simulink model "RainSnsrWiperMot_Method_1"  (R2021b)
settings: Solver=FixedStepDiscrete  StartTime=0.0  StopTime=10.0  FixedStep=0.01  RelTol=1e-3
undefined symbols (not defined in the file or in its folder): sigbuilder_block
libraries: simulink x1
settings Model: Creator=waleed.elshemy  LastModifiedBy=waleed.elshemy
settings OptimizationCC: DefaultParameterBehavior=Inlined  UseDivisionForNetSlopeComputation=on  GainParamInheritBuiltInType=on  UseFloatMulNetSlope=on  InlineInvariantSignals=on  PassReuseOutputArgsAs=Individual arguments  ZeroExternalMemoryAtStartup=off  ZeroInternalMemoryAtStartup=off  NoFixptDivByZeroProtection=on  EfficientFloat2IntCast=on  LifeSpan=1  OptimizeBlockOrder=speed  DifferentSizesBufferReuse=on  EfficientTunableParamExpr=on
settings DebuggingCC: ParameterTunabilityLossMsg=error
settings HardwareCC: ProdLongLongMode=on
settings SFSimCC: MATLABDynamicMemAlloc=off
settings RTWCC: Description=Embedded Coder  SystemTargetFile=ert.tlc  TemplateMakefile=ert_default_tmf
settings CodeAppCC: ForceParamTrailComments=on  IgnoreCustomStorageClasses=off  OperatorAnnotations=on  SimulinkDataObjDesc=on  SFDataObjDesc=on  CustomSymbolStrGlobalVar=rt$N$M  CustomSymbolStrType=$N$M  CustomSymbolStrFcn=$N$M$F  CustomSymbolStrMacro=$N$M  InsertBlockDesc=on
settings ERTTargetCC: TargetLangStandard=C99 (ISO)  GenerateSampleERTMain=on  IncludeMdlTerminateFcn=off  CombineSignalStateStructs=on  SupportComplex=off  SupportNonInlinedSFcns=on  InlinedParameterPlacement=NonHierarchical  ERTCustomFileTemplate=example_file_process.tlc  ERTFilePackagingFormat=CompactWithDataFile

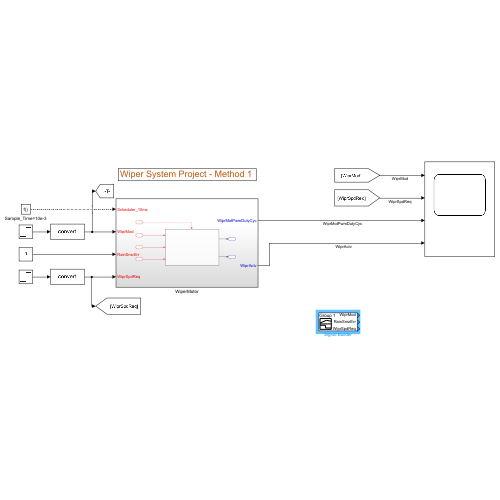
[thumbnail: Simulink's stored preview of the top-level diagram]
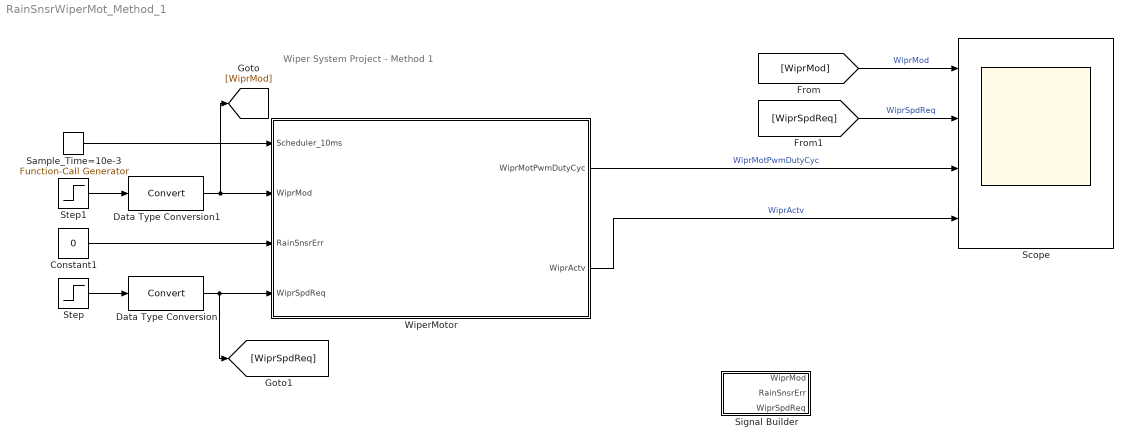
== system RainSnsrWiperMot_Method_1 ==
  note: Wiper System Project - Method 1
  Constant1 : Constant  Value=0  OutDataTypeStr=boolean
  Data Type Conversion : DataTypeConversion
  Data Type Conversion1 : DataTypeConversion
  Sample_Time=10e-3 : simulink/Ports & Subsystems/Function-Call Generator  sample_time=0.01  numberOfIterations=1  DisallowWideOutput=off
  Scope : Scope  NumInputPorts=4
  Signal Builder : Subsystem  Tag=STV Subsys  LoadFcn=sigbuilder_block('load');  StartFcn=sigbuilder_block('start');  StopFcn=sigbuilder_block('stop');  ClipboardFcn=sigbuilder_block('clipboard');  mask(Sigbuilder block){tuvar=[0:10]}
      mask help: Simulink:masks:SigbuilderBlock_MD
      mask init:
      | if ~strcmp(get_param(bdroot(gcbh),'SimulationStatus'),'stopped') tuvar = sigbuilder_block('maskInit'); end
      settings: CopyFcn=sigbuilder_block('copy');  DeleteFcn=sigbuilder_block('delete');  ModelCloseFcn=sigbuilder_block('modelClose');  PreSaveFcn=sigbuilder_block('preSave');  PauseFcn=sigbuilder_block('pause');  ContinueFcn=sigbuilder_block('continue');  NameChangeFcn=sigbuilder_block('namechange');  OpenFcn=sigbuilder_block('open',[404 117.5 550.5 362.5 ]);  CloseFcn=sigbuilder_block('close');
      mask Display: plot(0, 0, 100, 100,[2, 2, 32, 32, 2], [68, 8, 8, 68, 68],[32, 2], [38, 38], [32, 19, 2],[53, 60, 44], [32, 17, 17, 2],[16, 16, 31, 31]);txt = getActiveGroup(gcbh);text(2, 100, txt,'verticalAlignment', 'top');
  Step : Step  Time=3  Before=3  After=6  OutDataTypeStr=single
  Step1 : Step  Time=2  OutDataTypeStr=Inherit: Inherit via back propagation
  WiperMotor : Subsystem
  wires:
  Sample_Time=10e-3/1 -> WiperMotor/1(Scheduler_10ms)
  WiperMotor/1(WiprMotPwmDutyCyc) -> Scope/3  "WiprMotPwmDutyCyc"
  WiperMotor/2(WiprActv) -> Scope/4  "WiprActv"
  Step1/1 -> Data Type Conversion1/1
  Constant1/1 -> WiperMotor/3(RainSnsrErr)
  Step/1 -> Data Type Conversion/1
  Data Type Conversion/1 -> [WiprSpdReq], WiperMotor/4(WiprSpdReq)
  Data Type Conversion1/1 -> [WiprMod], WiperMotor/2(WiprMod)
  [WiprMod] -> Scope/1  "WiprMod"
  [WiprSpdReq] -> Scope/2  "WiprSpdReq"

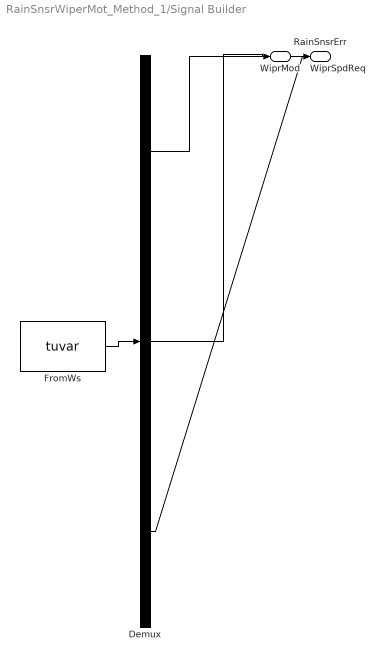
== system RainSnsrWiperMot_Method_1/Signal Builder ==
  Demux : Demux  Tag=STV Demux  Outputs=3
      settings: DisplayOption=none
  FromWs : FromWorkspace  Tag=STV FromWs  VariableName=tuvar  SampleTime=1  OutputAfterFinalValue=Holding final value
      SigBuilderData=|
      | common.afterFinalStr = 'Hold final value'
      | common.sampleTime = '1'
      | dataSet.timeRange = [0 16]
      | dataSet.name = 'Sheet1'
      | sbobj.Groups.Name = 'Sheet1'
      | sbobj.Groups.Signals(1).Name = 'WiprMod'
      | sbobj.Groups.Signals(1).XData = [0 1 2 3 4 5 6 7 8 9 10 11 12 13 14 15 16]
      | sbobj.Groups.Signals(1).YData = [0 0 2 2 3 3 1 1 1 1 1 1 1 1 1 1 1]
      | sbobj.Groups.Signals(2).Name = 'RainSnsrErr'
      | sbobj.Groups.Signals(2).XData = [0 1 2 3 4 5 6 7 8 9 10 11 12 13 14 15 16]
      | sbobj.Groups.Signals(2).YData = [0 0 0 0 0 0 0 0 0 0 0 0 0 0 0 1 0]
      | sbobj.Groups.Signals(3).Name = 'WiprSpdReq'
      | sbobj.Groups.Signals(3).XData = [0 1 2 3 4 5 6 7 8 9 10 11 12 13 14 15 16]
      | sbobj.Groups.Signals(3).YData = [0 0 0 0 0 0 0 0 1 2 3 4 5 6 7 7 7]
      | sbobj.Groups.TimeRange = [0 16]
  WiprMod : Outport  Tag=STV Outport
  RainSnsrErr : Outport  Tag=STV Outport  Port=2
  WiprSpdReq : Outport  Tag=STV Outport  Port=3
  wires:
  Demux/1 -> WiprMod/1
  FromWs/1 -> Demux/1
  Demux/2 -> RainSnsrErr/1
  Demux/3 -> WiprSpdReq/1

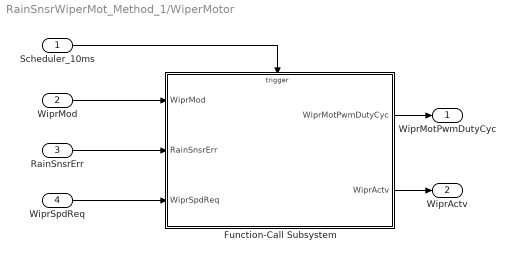
== system RainSnsrWiperMot_Method_1/WiperMotor ==
  Scheduler_10ms : Inport
  WiprMod : Inport  Port=2  OutMin=0  OutMax=3  OutDataTypeStr=uint8
  RainSnsrErr : Inport  Port=3  OutMin=0  OutMax=1  OutDataTypeStr=boolean
  WiprSpdReq : Inport  Port=4  OutMin=0  OutMax=7  OutDataTypeStr=uint8
  Function-Call Subsystem : Subsystem  TreatAsAtomicUnit=on
  WiprMotPwmDutyCyc : Outport  OutMin=0  OutMax=1  OutDataTypeStr=single  LockScale=on
  WiprActv : Outport  Port=2  OutDataTypeStr=boolean
  wires:
  WiprMod/1 -> Function-Call Subsystem/1(WiprMod)
  WiprSpdReq/1 -> Function-Call Subsystem/3(WiprSpdReq)
  Function-Call Subsystem/2(WiprActv) -> WiprActv/1
  Scheduler_10ms/1 -> Function-Call Subsystem/Trigger
  RainSnsrErr/1 -> Function-Call Subsystem/2(RainSnsrErr)
  Function-Call Subsystem/1(WiprMotPwmDutyCyc) -> WiprMotPwmDutyCyc/1

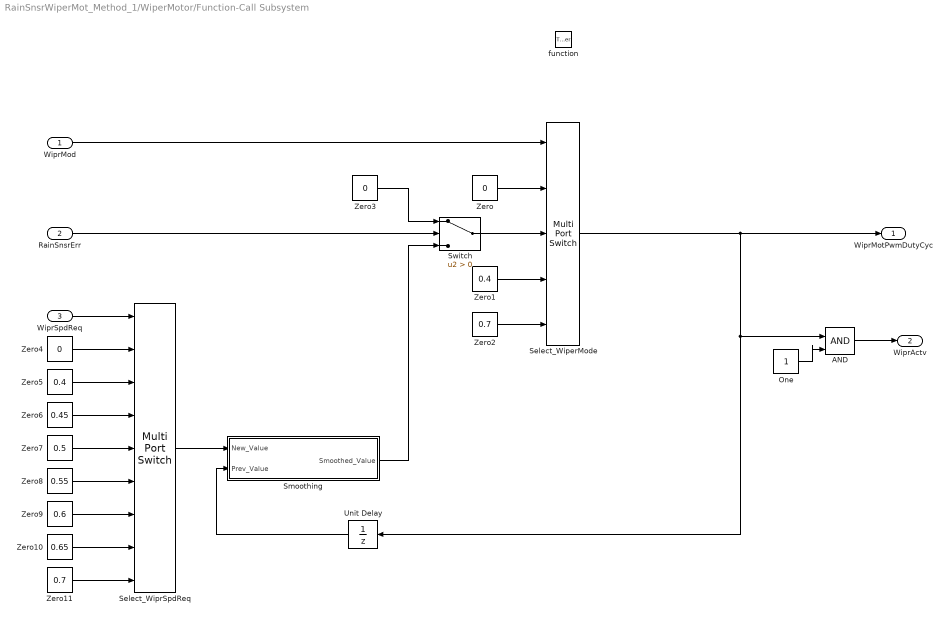
== system RainSnsrWiperMot_Method_1/WiperMotor/Function-Call Subsystem ==
  WiprMod : Inport
  RainSnsrErr : Inport  Port=2
  WiprSpdReq : Inport  Port=3
  function : TriggerPort  TriggerType=function-call  VariantControl=(inherit)
  AND : Logic  IconShape=distinctive  AllPortsSameDT=off  OutDataTypeStr=boolean
  One : Constant  OutDataTypeStr=Inherit: Inherit via back propagation
  Select_WiperMode : MultiPortSwitch  DataPortOrder=Zero-based contiguous  Inputs=4  zeroidx=on  OutDataTypeStr=single
  Select_WiprSpdReq : MultiPortSwitch  DataPortOrder=Zero-based contiguous  Inputs=8  zeroidx=on
  Smoothing : Subsystem
  Switch : Switch  Criteria=u2 > Threshold  OutDataTypeStr=single
  Unit Delay : UnitDelay  SampleTime=-1  HasFrameUpgradeWarning=on
  Zero : Constant  Value=0  OutDataTypeStr=Inherit: Inherit via back propagation
  Zero1 : Constant  Value=0.4  OutDataTypeStr=Inherit: Inherit via back propagation
  Zero10 : Constant  Value=0.65  OutDataTypeStr=Inherit: Inherit via back propagation
  Zero11 : Constant  Value=0.7  OutDataTypeStr=Inherit: Inherit via back propagation
  Zero2 : Constant  Value=0.7  OutDataTypeStr=Inherit: Inherit via back propagation
  Zero3 : Constant  Value=0  OutDataTypeStr=Inherit: Inherit via back propagation
  Zero4 : Constant  Value=0  OutDataTypeStr=Inherit: Inherit via back propagation
  Zero5 : Constant  Value=0.4  OutDataTypeStr=Inherit: Inherit via back propagation
  Zero6 : Constant  Value=0.45  OutDataTypeStr=Inherit: Inherit via back propagation
  Zero7 : Constant  Value=0.5  OutDataTypeStr=Inherit: Inherit via back propagation
  Zero8 : Constant  Value=0.55  OutDataTypeStr=Inherit: Inherit via back propagation
  Zero9 : Constant  Value=0.6  OutDataTypeStr=Inherit: Inherit via back propagation
  WiprMotPwmDutyCyc : Outport
  WiprActv : Outport  Port=2
  wires:
  WiprMod/1 -> Select_WiperMode/1
  Zero/1 -> Select_WiperMode/2
  Zero1/1 -> Select_WiperMode/4
  Zero2/1 -> Select_WiperMode/5
  Switch/1 -> Select_WiperMode/3
  RainSnsrErr/1 -> Switch/2
  Zero3/1 -> Switch/1
  Zero6/1 -> Select_WiprSpdReq/4
  Zero10/1 -> Select_WiprSpdReq/8
  Zero9/1 -> Select_WiprSpdReq/7
  WiprSpdReq/1 -> Select_WiprSpdReq/1
  Zero11/1 -> Select_WiprSpdReq/9
  Zero4/1 -> Select_WiprSpdReq/2
  Zero8/1 -> Select_WiprSpdReq/6
  Zero5/1 -> Select_WiprSpdReq/3
  Zero7/1 -> Select_WiprSpdReq/5
  Select_WiprSpdReq/1 -> Smoothing/1(New_Value)
  Select_WiperMode/1 -> Unit Delay/1, AND/1, WiprMotPwmDutyCyc/1
  AND/1 -> WiprActv/1
  Smoothing/1(Smoothed_Value) -> Switch/3
  Unit Delay/1 -> Smoothing/2(Prev_Value)
  One/1 -> AND/2

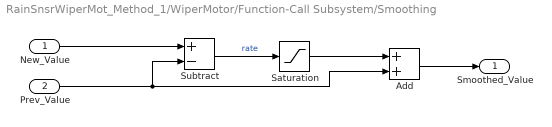
== system RainSnsrWiperMot_Method_1/WiperMotor/Function-Call Subsystem/Smoothing ==
  New_Value : Inport
  Prev_Value : Inport  Port=2
  Add : Sum
  Saturation : Saturate  UpperLimit=0.005  LowerLimit=-0.005
  Subtract : Sum  Inputs=+-
  Smoothed_Value : Outport
  wires:
  Prev_Value/1 -> Subtract/2, Add/2
  New_Value/1 -> Subtract/1
  Subtract/1 -> Saturation/1  "rate"
  Add/1 -> Smoothed_Value/1
  Saturation/1 -> Add/1
